simulink library "Dampers_Axle3_Interconnected"  (R2025a)
settings: Solver=VariableStepAuto  StartTime=0.0  StopTime=10.0  RelTol=1e-3
libraries: Damper_LeftRight x3
Description:
  | Component of Simscape Vehicle Templates Library
  | 
  | Copyright 2018-2025 The MathWorks, Inc.
settings Model: Creator=smiller  LastModifiedBy=smiller
settings SolverCC: AlgebraicLoopSolver=TrustRegion
settings DataIOCC: ReturnWorkspaceOutputs=off
settings OptimizationCC: ReuseModelBlockBuffer=off
settings DebuggingCC: UnconnectedInputMsg=warning  UnconnectedOutputMsg=warning  UnconnectedLineMsg=warning  ArithmeticOperatorsInVariantConditions=warning
settings ModelReferenceCC: EnableRefExpFcnMdlSchedulingChecks=on
settings SFSimCC: CustomCodeUndefinedFunction=UseInterfaceOnly
settings RTWCC: GPUComputeCapability=3.5  DLArmComputeVersion=19.05

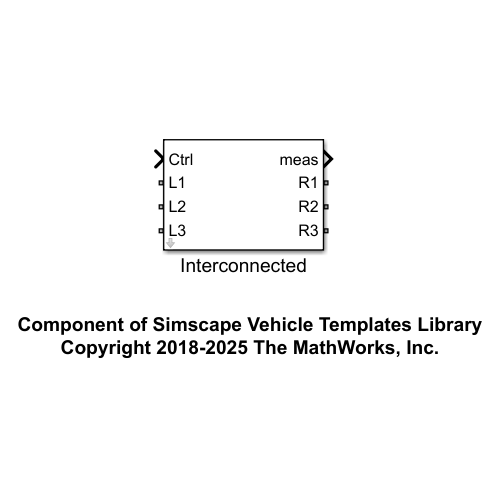
[thumbnail: Simulink's stored preview of the top-level diagram]
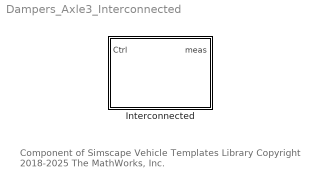
== system Dampers_Axle3_Interconnected ==
  note: Component of Simscape Vehicle Templates Library
      | Copyright 2018-2025 The MathWorks, Inc.
  Interconnected : Subsystem  VariantControl=Interconnected  mask(Interconnected Dampers){}
      mask help: Dampers connected across an axle.

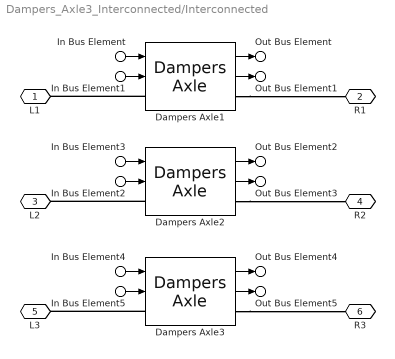
== system Dampers_Axle3_Interconnected/Interconnected ==
  In Bus Element1 : Inport  PortName=Ctrl  Element=R1
  In Bus Element : Inport  PortName=Ctrl  Element=L1
  In Bus Element3 : Inport  PortName=Ctrl  Element=L2
  In Bus Element2 : Inport  PortName=Ctrl  Element=R2
  In Bus Element4 : Inport  PortName=Ctrl  Element=L3
  In Bus Element5 : Inport  PortName=Ctrl  Element=R3
  Dampers Axle1 : Damper_LeftRight/Dampers Axle  VariantControl=Variant1  LabelModeActiveChoice=Linear  Damper=Damper.Axle1  VariantLabel=Damper.Axle1.class.Value
      settings: AttributesFormatString=%<ActiveVariant>
  Dampers Axle2 : Damper_LeftRight/Dampers Axle  VariantControl=Variant1  LabelModeActiveChoice=Linear  Damper=Damper.Axle2  VariantLabel=Damper.Axle2.class.Value
      settings: AttributesFormatString=%<ActiveVariant>
  Dampers Axle3 : Damper_LeftRight/Dampers Axle  VariantControl=Variant1  LabelModeActiveChoice=Linear  Damper=Damper.Axle3  VariantLabel=Damper.Axle3.class.Value
      settings: AttributesFormatString=%<ActiveVariant>
  L1 : PMIOPort  Side=Left
  R1 : PMIOPort  Port=2  Side=Right
  L2 : PMIOPort  Port=3  Side=Left
  R2 : PMIOPort  Port=4  Side=Right
  L3 : PMIOPort  Port=5  Side=Left
  R3 : PMIOPort  Port=6  Side=Right
  Out Bus Element : Outport  VectorParamsAs1DForOutWhenUnconnected=off  PortName=meas  Element=L1
  Out Bus Element1 : Outport  VectorParamsAs1DForOutWhenUnconnected=off  PortName=meas  Element=R1
  Out Bus Element2 : Outport  VectorParamsAs1DForOutWhenUnconnected=off  PortName=meas  Element=L2
  Out Bus Element3 : Outport  VectorParamsAs1DForOutWhenUnconnected=off  PortName=meas  Element=R2
  Out Bus Element4 : Outport  VectorParamsAs1DForOutWhenUnconnected=off  PortName=meas  Element=L3
  Out Bus Element5 : Outport  VectorParamsAs1DForOutWhenUnconnected=off  PortName=meas  Element=R3
  wires:
  Dampers Axle2/1 -> Out Bus Element2/1
  Dampers Axle2/2 -> Out Bus Element3/1
  In Bus Element2/1 -> Dampers Axle2/2
  In Bus Element3/1 -> Dampers Axle2/1
  Dampers Axle1/2 -> Out Bus Element1/1
  Dampers Axle1/1 -> Out Bus Element/1
  In Bus Element1/1 -> Dampers Axle1/2
  In Bus Element/1 -> Dampers Axle1/1
  In Bus Element4/1 -> Dampers Axle3/1
  In Bus Element5/1 -> Dampers Axle3/2
  Dampers Axle3/2 -> Out Bus Element5/1
  Dampers Axle3/1 -> Out Bus Element4/1
  connections:
  Dampers Axle1/RConn1 -- R1/RConn1
  Dampers Axle1/LConn1 -- L1/RConn1
  Dampers Axle2/RConn1 -- R2/RConn1
  Dampers Axle2/LConn1 -- L2/RConn1
  Dampers Axle3/LConn1 -- L3/RConn1
  Dampers Axle3/RConn1 -- R3/RConn1
